simulink model "analogicalgates_org"  (Simulink 10.0)
settings: Solver=ode45  StartTime=0.0  StopTime=10.0  RelTol=1e-3  EnableMultiTasking=on
settings Model: Creator=Elena  LastModifiedBy=annonymous
settings DataIOCC: LimitDataPoints=on
settings DebuggingCC: UnderspecifiedInitializationDetection=Simplified  MergeDetectMultiDrivingBlocksExec=error
settings GRTTargetCC: GeneratePreprocessorConditionals=Disable all  CombineOutputUpdateFcns=on  GRTInterface=off
settings ConfigComp: CovExternalEMLEnable=off

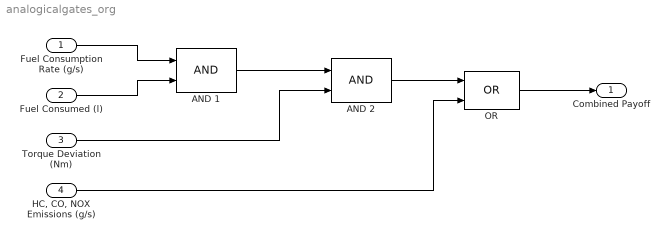
== system analogicalgates_org ==
  Fuel Consumption Rate (g/s) : Inport
  Fuel Consumed (l) : Inport  Port=2
  Torque Deviation (Nm) : Inport  Port=3
  "HC, CO, NOX Emissions (g/s)" : Inport  Port=4
  AND 1 : Logic  IconShape=distinctive  AllPortsSameDT=off  OutDataTypeStr=boolean
  AND 2 : Logic  IconShape=distinctive  AllPortsSameDT=off  OutDataTypeStr=boolean
  OR : Logic  Operator=OR  IconShape=distinctive  AllPortsSameDT=off  OutDataTypeStr=boolean
  Combined Payoff : Outport
  wires:
  Fuel Consumption Rate (g/s)/1 -> AND 1/1
  Fuel Consumed (l)/1 -> AND 1/2
  Torque Deviation (Nm)/1 -> AND 2/2
  AND 1/1 -> AND 2/1
  AND 2/1 -> OR/1
  "HC, CO, NOX Emissions (g/s)"/1 -> OR/2
  OR/1 -> Combined Payoff/1
